simulink model "Circuit_3RC_single_optimiser"  (R2024a)
settings: Solver=VariableStepAuto  StartTime=0.0  StopTime=stop_time  FixedStep=0.5  MaxStep=1  RelTol=1e-3
values from neighbouring files (symbols this model uses):
  C3 = tau3 ./ R3    [average_RC_parameters.m]    (also in optimise_RC_parameters.m = params(6) * scaling_factor_C3; pulse_sim.m = C3_charge)
  capacity = 115.8    [extract_R0.m]    (also in identify_pulses.m; optimise_RC_parameters.m = params(7); run_cell_sim.m)
  optimise_long = false    [optimise_RC_parameters.m]
  R0 = R0_charge    [optimise_RC_parameters.m]    (also in pulse_sim.m)
  R1 = params(1)    [optimise_RC_parameters.m]    (also in pulse_sim.m = R1_charge)
  R2 = params(3)    [optimise_RC_parameters.m]    (also in pulse_sim.m = R2_charge)
  R3 = params(5)    [optimise_RC_parameters.m]    (also in pulse_sim.m = R3_charge)
  soc_in = interp1(OCV.V(:, find(OCV.T == temperature)), OCV.SOC, actual_voltage_full.Data(1), "linear", 'extrap')    [optimise_RC_parameters.m]    (also in run_cell_sim.m = 1)
  temperature = 0    [average_RC_parameters.m]    (also in identify_pulses.m = temperature_data.Aux_CHTU1T__C_; optimise_RC_parameters.m = 45; pulse_sim.m; run_cell_sim.m = temperature_data.Aux_CHTU1T__C_)
undefined symbols (not defined in the file or in its folder): C3_from_optim, matrix, OCV, R3_from_optim
libraries: fl_lib x11, nesl_utility x8, ee_lib x1
settings Model: Creator=mmackenzie  LastModifiedBy=mmackenzie
settings OptimizationCC: ReuseModelBlockBuffer=off
settings RTWCC: GPUComputeCapability=3.5

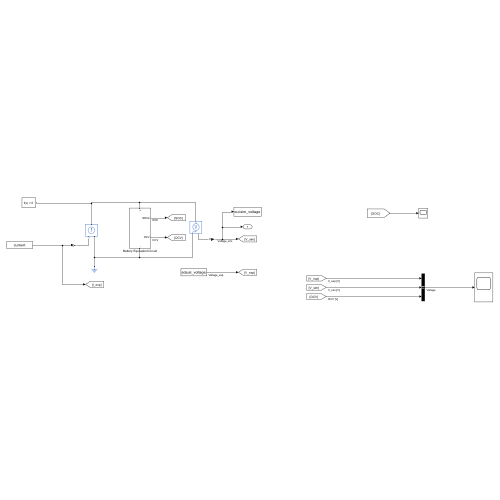
[thumbnail: Simulink's stored preview of the top-level diagram]
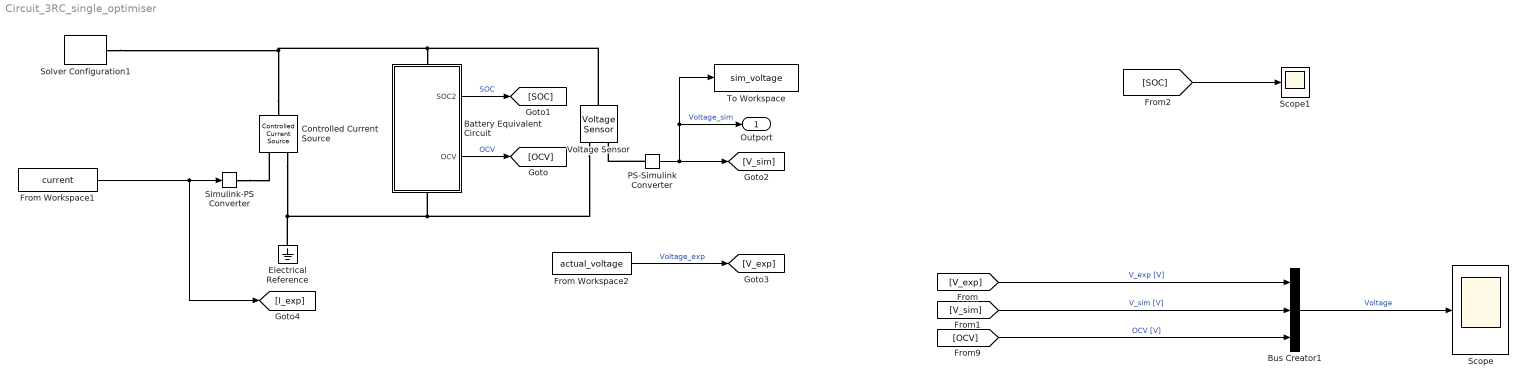
== system Circuit_3RC_single_optimiser ==
  Battery Equivalent Circuit : Subsystem
      settings: PortSchema="{\"entries\":[{\"content\":{\"sides\":[{\"content\":{\"connectorIds\":[]},\"type\":\"ConnectorPlacement.EquallySpacedRectSide\",\"uuid\":\"397b6d9d-31ba-4533-8816-c8a956765ed5\"},{\"content\":{\"connectorIds\":[\"Out1\",\"Out2\"],\"side\":\"RIGHT\"},\"type\":\"ConnectorPlacement.EquallySpacedRectSide\",\"uuid\":\"178b2ca9-d2d9-4380-91aa-f4497cccdf4f\"},{\"content\":{\"connectorIds\":[\"LConn1\"],\"side\":\"TOP\"},\"type\":\"ConnectorPlacement.EquallySpacedRectSide\",\"uuid\":\"4710d0ae-2920-4204-9cef-cbb5eb77e7ed\"},{\"content\":{\"connectorIds\":[\"RConn1\"],\"side\":\"BOTTOM\"},\"type\":\"ConnectorPlacement.EquallySpacedRectSide\",\"uuid\":\"673921ba-ed04-43cc-8806-353dbfb62c12\"}]},\"type\":\"ConnectorPlacement.EquallySpacedConnector\",\"uuid\":\"77ff7300-8565-4430-8966-d92537bdab4b\"}],\"packageUris\":[\"http://schema.mathworks.com/mf0/Connector/R2020b\"],\"version\":\"1.0\"}"
  Bus Creator1 : BusCreator  Inputs=3
  Controlled Current Source : fl_lib/Electrical/Electrical Sources/Controlled Current Source
  Electrical Reference : fl_lib/Electrical/Electrical Elements/Electrical Reference
  From Workspace1 : FromWorkspace  VariableName=current  SampleTime=0.5
  From Workspace2 : FromWorkspace  VariableName=actual_voltage  SampleTime=0.5
  PS-Simulink Converter : nesl_utility/PS-Simulink Converter  PhysicalDomain=network_engine_domain  SubClassName=ps_output  LeftPortType=input  RightPortType=output  PseudoPeriodic=off  Frequencies=[]  VectorFormat=inherit  Unit=inherit  AffineConversion=off
  Scope : Scope
  Scope1 : Scope
  Simulink-PS Converter : nesl_utility/Simulink-PS Converter  PhysicalDomain=network_engine_domain  SubClassName=ps_input  LeftPortType=input  RightPortType=output  PseudoPeriodic=off  Frequencies=[]  NoiseDistribution=none  NoiseParameters=[]  Unit=1  AffineConversion=off  FilteringAndDerivatives=provide  SimscapeFilterOrder=1  InputFilterTimeConstant=0.001  UdotUserProvided=0
  Solver Configuration1 : nesl_utility/Solver Configuration  PhysicalDomain=network_engine_domain  SubClassName=solver  LeftPortType=input  RightPortType=generic  Tones=[]  Harmonics=[]  SimulateNoise=off  Profile=off  UseLocalSampling=off  EnableSwitchedLinearOptims=on  FrequencyDomain=off  UseCCode=off  RelTol=0.001  AbsTol=0.001  MinStep=1e-09  ToWorkspace=off  RevertToSquareIcSolve=off  NumHomotopyIterations=100  PhasorMode=off  PhasorModeNumHarmonics=1  ConsistencySolver=NEWTON_FTOL  IndexReductionMethod=DerivativeReplacement  DoDC=off  ResidualTolerance=1e-09  ConsistencyTolSource=GLOBAL  ConsistencyAbsTol=0.001  ConsistencyRelTol=0.001  ConsistencyTolFactor=0.001  UseLocalSolver=off  LocalSolverChoice=NE_BACKWARD_EULER_ADVANCER  ResolveIndetEquations=on  FunctionEvalNumThread=1  LocalSolverSampleTime=0.001  DoFixedCost=off  MaxNonlinIter=3  MaxModeIter=2  ComputeImpulses=off  ImpulseIterations=2  LinearAlgebra=auto  LinearAlgebraNumThread=0  EquationFormulation=NE_TIME_EF  DelaysMemoryBudget=1024  AutomaticFiltering=on  FilteringTimeConstant=0.001  PartitionStorageMethod=AS_NEEDED  PartitionMemoryBudget=1024  PartitionMethod=ROBUST  MultibodyUseLocalSolver=off  MultibodyLocalSolverChoice=ODE1  MultibodyLocalSolverSampleTime=0.001
  To Workspace : ToWorkspace  VariableName=sim_voltage  SampleTime=-1
      settings: Save2DSignal=2-D array (concatenate along first dimension)
  Voltage Sensor : fl_lib/Electrical/Electrical Sensors/Voltage Sensor
  Outport : Outport
  wires:
  Battery Equivalent Circuit/1(SOC2) -> [SOC]  "SOC"
  Battery Equivalent Circuit/2(OCV) -> [OCV]  "OCV"
  From Workspace2/1 -> [V_exp]  "Voltage_exp"
  PS-Simulink Converter/1 -> To Workspace/1, Outport/1, [V_sim]  "Voltage_sim"
  [V_exp] -> Bus Creator1/1  "V_exp [V]"
  Bus Creator1/1 -> Scope/1  "Voltage"
  [V_sim] -> Bus Creator1/2  "V_sim [V]"
  [OCV] -> Bus Creator1/3  "OCV [V]"
  [SOC] -> Scope1/1
  From Workspace1/1 -> [I_exp], Simulink-PS Converter/1
  connections:
  Controlled Current Source/LConn1 -- Voltage Sensor/LConn1 -- Battery Equivalent Circuit/LConn1 -- Solver Configuration1/RConn1
  Electrical Reference/LConn1 -- Battery Equivalent Circuit/RConn1 -- Voltage Sensor/RConn2 -- Controlled Current Source/RConn2
  Simulink-PS Converter/RConn1 -- Controlled Current Source/RConn1
  PS-Simulink Converter/LConn1 -- Voltage Sensor/RConn1

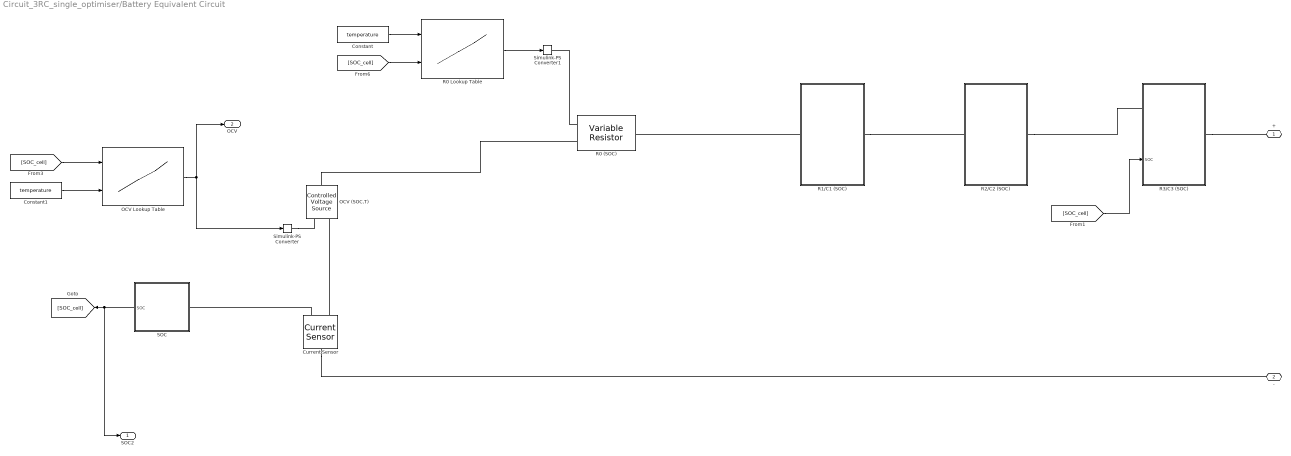
== system Circuit_3RC_single_optimiser/Battery Equivalent Circuit ==
  Constant : Constant  Value=temperature
  Constant1 : Constant  Value=temperature
  Current Sensor : fl_lib/Electrical/Electrical Sensors/Current Sensor
  OCV (SOC,T) : fl_lib/Electrical/Electrical Sources/Controlled Voltage Source
  OCV Lookup Table : Lookup_n-D  BreakpointsForDimension1=OCV.SOC  BreakpointsForDimension2=OCV.T  Table=OCV.V  ExtrapMethod=Clip  UseLastTableValue=on  InternalRulePriority=Speed  RndMeth=Simplest
      settings: InputPortMap=u0,u1
  R0 (SOC) : fl_lib/Electrical/Electrical Elements/Variable Resistor  Rmin=0 Ohm  thermalEnable=false  thermal_mass=1 J/K  i_specify=off  i_priority=None  i=0 A  i_nominal_specify=off  i_nominal_value=1  i_nominal_unit=A  v_specify=off  v_priority=None  v=0 V  v_nominal_specify=off  v_nominal_value=1  v_nominal_unit=V  T_specify=off  T_priority=None  T=300 K  T_nominal_specify=off  T_nominal_value=1  T_nominal_unit=K
  R0 Lookup Table : Lookup_n-D  BreakpointsForDimension1=R0.T  BreakpointsForDimension2=R0.SOC  Table=R0.R  ExtrapMethod=Clip  UseLastTableValue=on  InternalRulePriority=Speed  RndMeth=Simplest
      settings: InputPortMap=u0,u1
  R1/C1 (SOC) : Subsystem
  R2/C2 (SOC) : Subsystem
  R3/C3 (SOC) : Subsystem
      settings: PortSchema="{\"entries\":[{\"content\":{\"sides\":[{\"content\":{\"connectorIds\":[\"LConn1\",\"In1\"]},\"type\":\"ConnectorPlacement.EquallySpacedRectSide\",\"uuid\":\"c316f4d5-4ee3-4f31-94ae-630db377ee57\"},{\"content\":{\"connectorIds\":[\"RConn1\"],\"side\":\"RIGHT\"},\"type\":\"ConnectorPlacement.EquallySpacedRectSide\",\"uuid\":\"290ce4a0-a5ae-4ffa-bce5-68eaebe420b2\"},{\"content\":{\"connectorIds\":[],\"side\":\"TOP\"},\"type\":\"ConnectorPlacement.EquallySpacedRectSide\",\"uuid\":\"08b301c6-737b-4c96-90d5-35c84b053e01\"}]},\"type\":\"ConnectorPlacement.EquallySpacedConnector\",\"uuid\":\"3d3f4144-830a-466b-8a6c-edee7622600d\"}],\"packageUris\":[\"http://schema.mathworks.com/mf0/Connector/R2020b\"],\"version\":\"1.0\"}"
  SOC : Subsystem
      settings: PortSchema="{\"entries\":[{\"content\":{\"sides\":[{\"content\":{\"connectorIds\":[\"Out1\"]},\"type\":\"ConnectorPlacement.EquallySpacedRectSide\",\"uuid\":\"7d8ebd59-8052-4308-b26c-7ff9f1f69d1b\"},{\"content\":{\"connectorIds\":[\"RConn1\"],\"side\":\"RIGHT\"},\"type\":\"ConnectorPlacement.EquallySpacedRectSide\",\"uuid\":\"c18676c0-c2b9-46af-80cc-bb3d6a3fac14\"},{\"content\":{\"connectorIds\":[],\"side\":\"TOP\"},\"type\":\"ConnectorPlacement.EquallySpacedRectSide\",\"uuid\":\"047d6f7f-9f32-4229-9b30-4a4b1fb31892\"}]},\"type\":\"ConnectorPlacement.EquallySpacedConnector\",\"uuid\":\"faef4339-4ab6-438f-b9c7-b924a206f9a5\"}],\"packageUris\":[\"http://schema.mathworks.com/mf0/Connector/R2020b\"],\"version\":\"1.0\"}"
  Simulink-PS Converter : nesl_utility/Simulink-PS Converter  PhysicalDomain=network_engine_domain  SubClassName=ps_input  LeftPortType=input  RightPortType=output  PseudoPeriodic=off  Frequencies=[]  NoiseDistribution=none  NoiseParameters=[]  Unit=1  AffineConversion=off  FilteringAndDerivatives=provide  SimscapeFilterOrder=1  InputFilterTimeConstant=0.001  UdotUserProvided=0
  Simulink-PS Converter1 : nesl_utility/Simulink-PS Converter  PhysicalDomain=network_engine_domain  SubClassName=ps_input  LeftPortType=input  RightPortType=output  PseudoPeriodic=off  Frequencies=[]  NoiseDistribution=none  NoiseParameters=[]  Unit=1  AffineConversion=off  FilteringAndDerivatives=provide  SimscapeFilterOrder=1  InputFilterTimeConstant=0.001  UdotUserProvided=0
  + : PMIOPort  Side=Left
  - : PMIOPort  Port=2  Side=Right
  SOC2 : Outport
  OCV : Outport  Port=2
  wires:
  SOC/1(SOC) -> SOC2/1, [SOC_cell]
  [SOC_cell] -> R3/C3 (SOC)/1(SOC)
  [SOC_cell] -> R0 Lookup Table/2
  R0 Lookup Table/1 -> Simulink-PS Converter1/1
  Constant/1 -> R0 Lookup Table/1
  Constant1/1 -> OCV Lookup Table/2
  OCV Lookup Table/1 -> Simulink-PS Converter/1, OCV/1
  [SOC_cell] -> OCV Lookup Table/1
  connections:
  Current Sensor/RConn1 -- SOC/RConn1
  Simulink-PS Converter/RConn1 -- OCV (SOC,T)/RConn1
  Current Sensor/LConn1 -- -/RConn1
  Current Sensor/RConn2 -- OCV (SOC,T)/RConn2
  OCV (SOC,T)/LConn1 -- R0 (SOC)/LConn2
  R1/C1 (SOC)/RConn1 -- R2/C2 (SOC)/LConn1
  R3/C3 (SOC)/RConn1 -- +/RConn1
  R1/C1 (SOC)/LConn1 -- R0 (SOC)/RConn1
  R2/C2 (SOC)/RConn1 -- R3/C3 (SOC)/LConn1
  R0 (SOC)/LConn1 -- Simulink-PS Converter1/RConn1

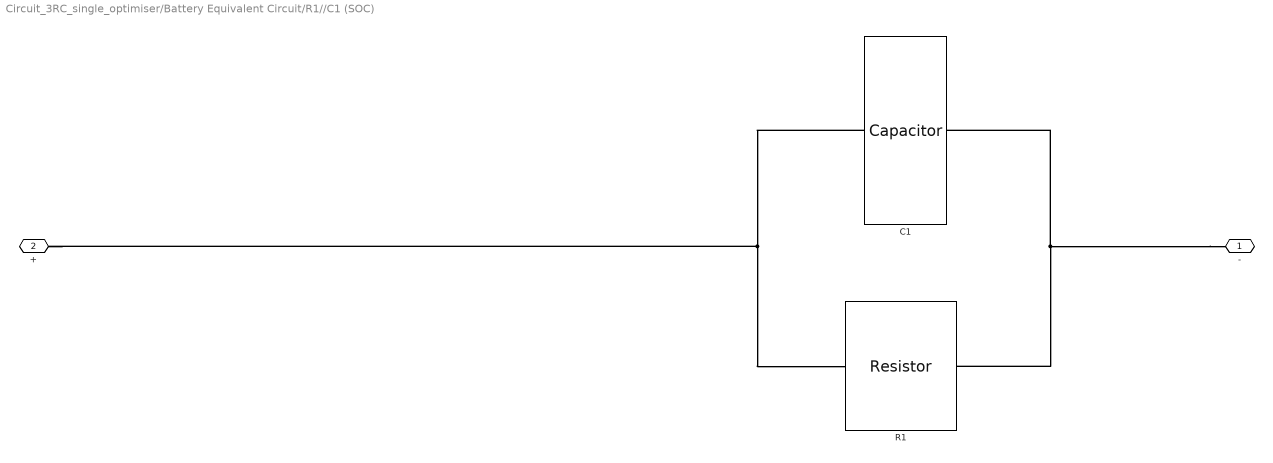
== system Circuit_3RC_single_optimiser/Battery Equivalent Circuit/R1//C1 (SOC) ==
  C1 : fl_lib/Electrical/Electrical Elements/Capacitor  c=C1 F  r=1e-6 Ohm  g=0 1/Ohm  i_specify=off  i_priority=None  i=0 A  i_nominal_specify=off  i_nominal_value=1  i_nominal_unit=A  v_specify=off  v_priority=None  v=0 V  v_nominal_specify=off  v_nominal_value=1  v_nominal_unit=V  vc_specify=off  vc_priority=High  vc=0 V  vc_nominal_specify=off  vc_nominal_value=1  vc_nominal_unit=V
  R1 : fl_lib/Electrical/Electrical Elements/Resistor  R=R1 Ohm  i_specify=off  i_priority=None  i=0 A  i_nominal_specify=off  i_nominal_value=1  i_nominal_unit=A  v_specify=off  v_priority=None  v=0 V  v_nominal_specify=off  v_nominal_value=1  v_nominal_unit=V
  - : PMIOPort  Side=Right
  + : PMIOPort  Port=2  Side=Left
  connections:
  +/RConn1 -- R1/LConn1 -- C1/LConn1
  -/RConn1 -- R1/RConn1 -- C1/RConn1

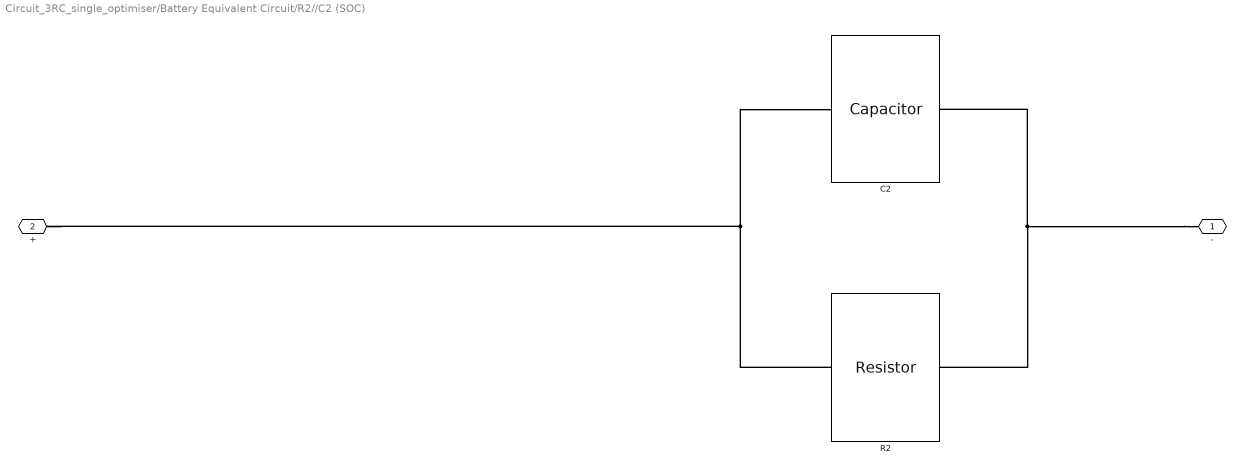
== system Circuit_3RC_single_optimiser/Battery Equivalent Circuit/R2//C2 (SOC) ==
  C2 : fl_lib/Electrical/Electrical Elements/Capacitor  c=C2 F  r=1e-6 Ohm  g=0 1/Ohm  i_specify=off  i_priority=None  i=0 A  i_nominal_specify=off  i_nominal_value=1  i_nominal_unit=A  v_specify=off  v_priority=None  v=0 V  v_nominal_specify=off  v_nominal_value=1  v_nominal_unit=V  vc_specify=off  vc_priority=High  vc=0 V  vc_nominal_specify=off  vc_nominal_value=1  vc_nominal_unit=V
  R2 : fl_lib/Electrical/Electrical Elements/Resistor  R=R2 Ohm  i_specify=off  i_priority=None  i=0 A  i_nominal_specify=off  i_nominal_value=1  i_nominal_unit=A  v_specify=off  v_priority=None  v=0 V  v_nominal_specify=off  v_nominal_value=1  v_nominal_unit=V
  - : PMIOPort  Side=Right
  + : PMIOPort  Port=2  Side=Left
  connections:
  -/RConn1 -- R2/RConn1 -- C2/RConn1
  +/RConn1 -- R2/LConn1 -- C2/LConn1

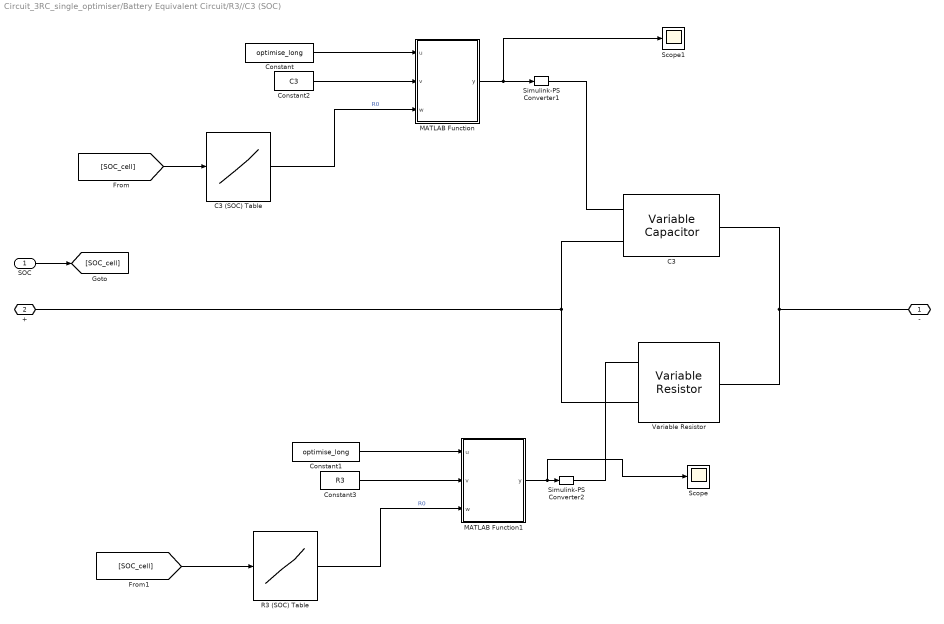
== system Circuit_3RC_single_optimiser/Battery Equivalent Circuit/R3//C3 (SOC) ==
  SOC : Inport
  C3 : ee_lib/Passive/Variable Capacitor  prm=2  Cmin=1e-9 F  r=1e-6 Ohm  v0=0 V  q0=0 C
      settings: InternalSimscapePortConfiguration="{\"Bottom\":[],\"Left\":[{\"id\":\"C\",\"label\":\"C\",\"type\":\"input\"},{\"id\":\"p\",\"label\":\"+\",\"type\":\"foundation.electrical.electrical\"}],\"Right\":[{\"id\":\"n\",\"label\":\"-\",\"type\":\"foundation.electrical.electrical\"}],\"Top\":[]}"
  C3 (SOC) Table : Lookup_n-D  NumberOfTableDimensions=1  BreakpointsForDimension1=C3_from_optim.SOC  BreakpointsForDimension2=unique(matrix.Temperatura)  BreakpointsForDimension3=[5, 7]  Table=C3_from_optim.C  ExtrapMethod=Clip  UseLastTableValue=on  InternalRulePriority=Speed  RndMeth=Simplest
  Constant : Constant  Value=optimise_long
  Constant1 : Constant  Value=optimise_long
  Constant2 : Constant  Value=C3
  Constant3 : Constant  Value=R3
  MATLAB Function : MATLAB Function  TreatAsAtomicUnit=on
  MATLAB Function1 : MATLAB Function  TreatAsAtomicUnit=on
  R3 (SOC) Table : Lookup_n-D  NumberOfTableDimensions=1  BreakpointsForDimension1=R3_from_optim.SOC  BreakpointsForDimension2=unique(matrix.Temperatura)  BreakpointsForDimension3=[5, 7]  Table=R3_from_optim.R  ExtrapMethod=Clip  UseLastTableValue=on  InternalRulePriority=Speed  RndMeth=Simplest
  Scope : Scope
  Scope1 : Scope
  Simulink-PS Converter1 : nesl_utility/Simulink-PS Converter  PhysicalDomain=network_engine_domain  SubClassName=ps_input  LeftPortType=input  RightPortType=output  PseudoPeriodic=off  Frequencies=[]  NoiseDistribution=none  NoiseParameters=[]  Unit=1  AffineConversion=off  FilteringAndDerivatives=provide  SimscapeFilterOrder=1  InputFilterTimeConstant=0.001  UdotUserProvided=0
  Simulink-PS Converter2 : nesl_utility/Simulink-PS Converter  PhysicalDomain=network_engine_domain  SubClassName=ps_input  LeftPortType=input  RightPortType=output  PseudoPeriodic=off  Frequencies=[]  NoiseDistribution=none  NoiseParameters=[]  Unit=1  AffineConversion=off  FilteringAndDerivatives=provide  SimscapeFilterOrder=1  InputFilterTimeConstant=0.001  UdotUserProvided=0
  Variable Resistor : fl_lib/Electrical/Electrical Elements/Variable Resistor  Rmin=0 Ohm  thermalEnable=false  thermal_mass=1 J/K  i_specify=off  i_priority=None  i=0 A  i_nominal_specify=off  i_nominal_value=1  i_nominal_unit=A  v_specify=off  v_priority=None  v=0 V  v_nominal_specify=off  v_nominal_value=1  v_nominal_unit=V  T_specify=off  T_priority=None  T=300 K  T_nominal_specify=off  T_nominal_value=1  T_nominal_unit=K
  - : PMIOPort  Side=Right
  + : PMIOPort  Port=2  Side=Left
  wires:
  Constant/1 -> MATLAB Function/1(u)
  Constant2/1 -> MATLAB Function/2(v)
  C3 (SOC) Table/1 -> MATLAB Function/3(w)  "R0"
  MATLAB Function/1(y) -> Scope1/1, Simulink-PS Converter1/1
  MATLAB Function1/1(y) -> Scope/1, Simulink-PS Converter2/1
  [SOC_cell] -> R3 (SOC) Table/1
  Constant1/1 -> MATLAB Function1/1(u)
  Constant3/1 -> MATLAB Function1/2(v)
  R3 (SOC) Table/1 -> MATLAB Function1/3(w)  "R0"
  SOC/1 -> [SOC_cell]
  [SOC_cell] -> C3 (SOC) Table/1
  connections:
  -/RConn1 -- Variable Resistor/RConn1 -- C3/RConn1
  +/RConn1 -- Variable Resistor/LConn2 -- C3/LConn2
  Simulink-PS Converter2/RConn1 -- Variable Resistor/LConn1
  Simulink-PS Converter1/RConn1 -- C3/LConn1

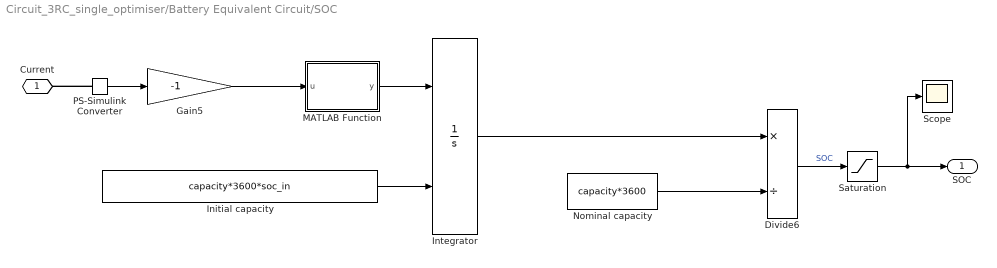
== system Circuit_3RC_single_optimiser/Battery Equivalent Circuit/SOC ==
  Divide6 : Product  Inputs=*/  RndMeth=Zero  SaturateOnIntegerOverflow=on
  Gain5 : Gain  Gain=-1
  Initial capacity : Constant  Value=capacity*3600*soc_in
  Integrator : Integrator  InitialConditionSource=external  IgnoreLimit=on  ZeroCross=off
  MATLAB Function : MATLAB Function  TreatAsAtomicUnit=on
  Nominal capacity : Constant  Value=capacity*3600
  PS-Simulink Converter : nesl_utility/PS-Simulink Converter  PhysicalDomain=network_engine_domain  SubClassName=ps_output  LeftPortType=input  RightPortType=output  PseudoPeriodic=off  Frequencies=[]  VectorFormat=inherit  Unit=inherit  AffineConversion=off
  Saturation : Saturate  UpperLimit=1  LowerLimit=0
  Scope : Scope
  Current : PMIOPort  Side=Right
  SOC : Outport
  wires:
  Nominal capacity/1 -> Divide6/2
  Integrator/1 -> Divide6/1
  Initial capacity/1 -> Integrator/2
  Gain5/1 -> MATLAB Function/1(u)
  Divide6/1 -> Saturation/1  "SOC"
  PS-Simulink Converter/1 -> Gain5/1
  Saturation/1 -> Scope/1, SOC/1
  MATLAB Function/1(y) -> Integrator/1
  connections:
  PS-Simulink Converter/LConn1 -- Current/RConn1

== matlab function Circuit_3RC_single_optimiser/Battery Equivalent Circuit/SOC/MATLAB Function ==
  data: u input; y output
function y = fcn(u)
if u>0
    y=0.99*u;
else
y = u;
end

== matlab function Circuit_3RC_single_optimiser/Battery Equivalent Circuit/R3//C3 (SOC)/MATLAB Function1 ==
  data: u input; y output; v input; w input
function y = fcn(u, v, w)
if u == 1
    y = v;
else
    y = w;
end

== matlab function Circuit_3RC_single_optimiser/Battery Equivalent Circuit/R3//C3 (SOC)/MATLAB Function ==
  data: u input; y output; v input; w input
function y = fcn(u, v, w)
if u == 1
    y = v;
else
    y = w;
end
